simulink library "UXFD_Lib"  (R2016b)
settings: Solver=ode45  StartTime=0.0  StopTime=10.0  RelTol=1e-3  EnableMultiTasking=on
undefined symbols (not defined in the file): BreakpointData, BreakpointData1, BreakpointData2, BreakpointData_One_A, BreakpointData_Two_A, E2E_P01DataIDMode, E2E_P01ReceiverStatusType, EnumClass, iBit, initalValue, No_Runnable_Period, ObB_EidBsgStDerat_C, p_OVERRIDE_MASTER_SWITCH, SlDemoSign, SwitchOff_P, SwitchOn_P, Table, TableData_M, VCCTi33, VSysD_FidVehDerat1_C
libraries: simulink x28, CCMLib x11, UXFD_Lib x8, canmsglib x2, PTCC_Lib x1, hdlsllib x1
(part 4 of 7)

== system UXFD_Lib/Standard/Discrete dynamics ==
  note: Hystresis filter
  note: Bumpless transfer
  note: Unit delay
  note: Discrete
      | derivate
  note: Rate limiter
  note: First order filters (VCC)
  note: Second order filters(VCC)
  BumplessRateTransfer : Subsystem  mask(VCC_BumplessTransferRate_1.0){}
      mask help:
      | Makes a bumpless rate transfer from u2  to u1
      | when s goes from 0 to 1. It is very important that
      |  the Trig signal assumes the values <= 0 and >= 1.
      | The transfer happens during a time controlled by a
      | filter with a time constant that can be calibrated.
      settings: CopyFcn=set_param(gcbh,'ShowName','off');
      mask Display:
      | plot([0.2 1], [0.2 0.2]);
      | plot([0.2 0.3], [0.22 0.22]);
      | plot([0.7 1], [0.78 0.78]);
      | plot([0.2 1], [0.8 0.8]);
      | plot([0.7 1], [0.78 0.78]);
      | plot([0.3 0.7],[0.22, 0.78])
      | plot([0.38, 0.5, 0.52], [0.46, 0.5, 0.37])
  BumplessTransfer : Subsystem  mask(GL_BumplessTransferFilter_1.0){}
      mask help:
      | Makes a bumpless transfer from u2  to u1
      | when s goes from 0 to 1. It is very important that
      |  the Trig signal assumes the values <= 0 and >= 1.
      | The transfer happens during a time controlled by a
      | filter with a time constant that can be calibrated.
      mask init:
      | set_param(gcb,'LinkStatus','none');
      settings: CopyFcn=set_param(gcbh,'ShowName','off');
      mask Display:
      | plot([0.15 1], [0.2 0.2]);
      | plot([0.15 1], [0.8 0.8]);
      | plot([0.00 0.50 1.00 1.50 2.00 2.50 3.00 ]/3*0.7+0.3, ...
      |      [0.20 0.52 0.67 0.74 0.77 0.79 0.79]);
      | 
      | plot([0.28, 0.4, 0.47], [0.48, 0.5, 0.42])
  DLPF1_pole_v2 : Subsystem  mask(GL_DiscreteDerivative_1.0){}
      mask help:
      | Discrete derivative and low-pass filter. Corresponding analogue transfer function:
      |   s / (1 + tc * s)
      mask init:
      | set_param(gcb,'LinkStatus','none');
      settings: CopyFcn=set_param(gcbh,'ShowName','off');
      mask Display:
      | plot([0.35, 0.9], [0, 0], [0.35, 0.35], [0, 1])
      | plot(0.35:0.55/10:0.9,  1- [0 0.39 0.63 0.78 0.86 0.92 0.95 0.97 0.98 0.99 0.99])
  FirstOrderFilter : Subsystem  mask(VCC_FirstOrderFilter_1.0){}
      mask help: Discrete low-pass filter. Corresponding analogue transfer function: 1 / (1 + tc * s)
      settings: CopyFcn=set_param(gcbh,'ShowName','on');
      mask Display:
      | plot([0.35, 0.9], [0, 0], [0.35, 0.35], [0, 1])
      | plot(0.35:0.55/10:0.9,   [0 0.39 0.63 0.78 0.86 0.92 0.95 0.98 0.99 0.99 0.99])
  FirstOrderFilter1 : Subsystem  mask(VCC_FirstOrderFilterExtraFeat_1.0){}
      mask help:
      | Discrete low-pass filter. Corresponding analogue transfer function: 1 / (1 + tc * s)
      |
      | Parameters:
      | Error - An output which shows the difference between the input and output signal values
      | Different increase and decrease tc -
      | Reset - Sets the output value = rv when r = 1
      settings: CopyFcn=set_param(gcbh,'ShowName','on');
      mask Display:
      | plot([0.35, 0.9], [0, 0], [0.35, 0.35], [0, 1])
      | plot(0.35:0.55/10:0.9,   [0 0.39 0.63 0.78 0.86 0.92 0.95 0.98 0.99 0.99 0.99])
  HysteresisFilter : Subsystem  mask(GL_HysteresisFilter_1.0){}
      mask help:
      | Filter to avoid occilation during low slipp
      | when converter character is steep
      mask init:
      | set_param(gcb,'LinkStatus','none');
      settings: CopyFcn=set_param(gcbh,'ShowName','off');
      mask Display:
      | text(0.1, 0.8, 'u');
      | text(0.1, 0.3, 'h');
      | plot([0.3, 0.6, 0.9], [0.1, 0.1, 0.9]);
      | plot([0.3, 0.6, 0.9], [0.1, 0.9, 0.9]);
      | plot([0.4, 0.55], [0.4, 0.4]);
      | plot([0.7, 0.84], [0.7, 0.7]);
  LPF1_discreteReset : Subsystem  Description=|  mask(PAG_FirstOrder_Smoothing_Filter_Reset_LV1.8_BV5){OpenTL=Select block:, OutputLineName=}
      | Purpose Use the block to implement a discrete low pass filter.
      | 
      | When the input signal r is TRUE the output will assume the
      | value of the input signal. This is used to set initial values of
      | the filter.
      | 
      | Difference to Simulink and justification
      | Additional block to perform special feature for ECM implementation
      | in a standard manner. Block name hidden, since icon clearly conveys
      | meaning and name adds unnecessary clutter to the page.
      mask prompts: OpenTL "Open Target Link dialog"; OutputLineName "Output line name"
      mask help:
      | Discrete first order low pass filter. Discrete transfer function:
      | y(k)=a*y(k-1)+(1-a)*u(k)
      | When the input signal r is TRUE the output will assume the
      | value of the input signal. This is used to set initial values of
      | the filter.
      mask init:
      | %% Reset the opendialog popupvalue
      | Values=get_param(gcbh,'maskvalues');
      | Values{1}='Select block:';
      | set_param(gcbh,'maskvalues',Values);
      | 
      | %Set the line name, 
      | CurrentBlock=gcbh;
      | %Find the output variable block
      | while strcmp(get_param(CurrentBlock,'blocktype'),'SubSystem')
      |     Tmp=get_param(find_system(CurrentBlock,'lookundermasks','on','searchdepth',1,'blocktype','Outport','Port','1'),'linehandles');
      |     CurrentBlock=get_param(Tmp.Inport,'srcblockhandle');
      | end
      | set_param(Tmp.Inport,'name',get_param(gcbh,'OutputLineName'));
      | 
      | 
      | %% Adjust the propagated output line name
      | Tmp=get_param(gcbh,'linehandles');
      | OutputLine=Tmp.Outport;
      | if OutputLine~=-1
      |     
      |     if isempty(get_param(gcbh,'OutputLineName'))
      |         set(OutputLine,'signalPropagation','off')
      |         set(OutputLine,'name','')
      |     else
      |         set(OutputLine,'name',['<' get_param(gcbh,'OutputLineName') '>'])
      |     end
      | end
      settings: CopyFcn=set_param(gcbh,'ShowName','on');
      mask TypeOptions OpenTL: Select block: | Output variable
      mask Callback OpenTL:
      | if strcmp(get_param(gcbh,'OpenTL'),'Output variable')
      |     BlockType='SubSystem';
      |     OutputVariableBlock=gcbh;
      |     while strcmp(BlockType,'SubSystem');
      |     Tmp=get_param(find_system(OutputVariableBlock,'lookundermasks','on','searchdepth',1,'blocktype','Outport','Port','1'),'linehandles');
      |     OutputVariableBlock=get_param(Tmp.Inport,'srcblockhandle');
      |     BlockType=get_param(OutputVariableBlock,'blocktype');
      |     end
      | 
      |     MaskType=get_param(OutputVariableBlock,'masktype');
      |     if strmatch('TL',MaskType)
      | 
      |         if ismember(MaskType,{'TL_Sum','TL_Product'})
      |             MaskName='tl_sumprod_dlg';
      |         elseif ismember(MaskType,{'TL_LogicalOperator','TL_RelationalOperator'})
      |             MaskName='tl_rel_dlg';
      |         elseif strcmp(MaskType,'TL_MinMax')
      |             MaskName='tl_minmax_dlg';
      |         elseif strcmp(MaskType,'TL_Gain')
      |             MaskName='tl_gain_dlg';
      |         elseif strcmp(MaskType,'TL_Switch')
      |             MaskName='tl_switch_dlg';
      |         end
      | 
      |         dstabdlg('create',MaskName,OutputVariableBlock);
      |     end
      | end
      mask Display:
      | plot([0.3, 1], [0, 0], [0.3, 0.3], [0, 1])
      | plot([0 0.1 0.1 0.2 0.2 0.3 0.3 0.4 0.4 0.5 0.5 0.6 0.6 0.7 0.7 0.8 0.8 0.9 0.9 1 1]*0.7+0.3, [ 0 0 0.39 0.39 0.63 0.63 0.78 0.78 0.86 0.86 0.92 0.92 0.95 0.95 0.97 0.97 0.98 0.98 0.99 0.99 0.99])
  LPF2_discrete : Subsystem  mask(PAG_SecondOrder_Discrete_Filter_LV1.8_BV3){OpenTL=Select block:, OutputLineName=}
      mask prompts: OpenTL "Open Target Link dialog"; OutputLineName "Output line name"
      mask help:
      | Discrete  filter.
      |
      | y(k) = -a1 y(k-1) - a2 y(k-2) + b0 u(k) + b1 u(k-1) + b2 u(k-2)
      mask init: same as UXFD_Lib/Standard/Discrete dynamics/LPF1_discreteReset
      settings: CopyFcn=set_param(gcbh,'ShowName','off');
      mask TypeOptions OpenTL: Select block: | Output variable
      mask Callback OpenTL:
      | if strcmp(get_param(gcbh,'OpenTL'),'Output variable')
      |     BlockType='SubSystem';
      |     OutputVariableBlock=gcbh;
      |     while strcmp(BlockType,'SubSystem');
      |     Tmp=get_param(find_system(OutputVariableBlock,'lookundermasks','on','searchdepth',1,'blocktype','Outport','Port','1'),'linehandles');
      |     OutputVariableBlock=get_param(Tmp.Inport,'srcblockhandle');
      |     BlockType=get_param(OutputVariableBlock,'blocktype');
      |     end
      | 
      |     MaskType=get_param(OutputVariableBlock,'masktype');
      |     if strmatch('TL',MaskType)
      | 
      |         if ismember(MaskType,{'TL_Sum','TL_Product'})
      |             MaskName='tl_sumprod_dlg';
      |         elseif ismember(MaskType,{'TL_LogicalOperator','TL_RelationalOperator'})
      |             MaskName='tl_rel_dlg';
      |         elseif strcmp(MaskType,'TL_MinMax')
      |             MaskName='tl_minmax_dlg';
      |         elseif strcmp(MaskType,'TL_Gain')
      |             MaskName='tl_gain_dlg';
      |         elseif strcmp(MaskType,'TL_Switch')
      |             MaskName='tl_switch_dlg';
      |         end
      | 
      |         dstabdlg('create',MaskName,OutputVariableBlock);
      |     end
      | end
      mask Display:
      | plot([0.45, 1], [0, 0], [0.45, 0.45], [0, 1])
      | plot([0 0.1 0.1 0.2 0.2 0.3 0.3 0.4 0.4 0.5 0.5 0.6 0.6 0.7 0.7 0.8 0.8 0.9 0.9 1 1]*0.55+0.45, [ 0 0 0.39 0.39 0.63 0.63 0.78 0.78 0.86 0.86 0.92 0.92 0.95 0.95 0.97 0.97 0.98 0.98 0.99 0.99 0.99])
  LPF2_omega : Subsystem  mask(PAG_SecondOrder_Filter_LV1.8_BV4){OpenTL=Select block:, OutputLineName=}
      mask prompts: OpenTL "Open Target Link dialog"; OutputLineName "Output line name"
      mask help:
      | An Euler discretization of a filter with transfer function
      |                          2
      |                       w
      | G(s) = -----------------------------
      |              2                     2
      |            s  + 2 w z s + w
      mask init: same as UXFD_Lib/Standard/Discrete dynamics/LPF1_discreteReset
      settings: CopyFcn=set_param(gcbh,'ShowName','off');
      mask TypeOptions OpenTL: Select block: | Output variable
      mask Callback OpenTL:
      | if strcmp(get_param(gcbh,'OpenTL'),'Output variable')
      |     BlockType='SubSystem';
      |     OutputVariableBlock=gcbh;
      |     while strcmp(BlockType,'SubSystem');
      |     Tmp=get_param(find_system(OutputVariableBlock,'lookundermasks','on','searchdepth',1,'blocktype','Outport','Port','1'),'linehandles');
      |     OutputVariableBlock=get_param(Tmp.Inport,'srcblockhandle');
      |     BlockType=get_param(OutputVariableBlock,'blocktype');
      |     end
      | 
      |     MaskType=get_param(OutputVariableBlock,'masktype');
      |     if strmatch('TL',MaskType)
      | 
      |         if ismember(MaskType,{'TL_Sum','TL_Product'})
      |             MaskName='tl_sumprod_dlg';
      |         elseif ismember(MaskType,{'TL_LogicalOperator','TL_RelationalOperator'})
      |             MaskName='tl_rel_dlg';
      |         elseif strcmp(MaskType,'TL_MinMax')
      |             MaskName='tl_minmax_dlg';
      |         elseif strcmp(MaskType,'TL_Gain')
      |             MaskName='tl_gain_dlg';
      |         elseif strcmp(MaskType,'TL_Switch')
      |             MaskName='tl_switch_dlg';
      |         end
      | 
      |         dstabdlg('create',MaskName,OutputVariableBlock);
      |     end
      | end
      mask Display:
      | plot([0.45, 0.9], [0, 0], [0.45, 0.45], [0, 1])
      | plot(0.45:0.45/10:0.9,   [ 0 0.05 0.1 0.8 1.0 0.95 0.85 0.9 0.95 0.92 0.9 ])
  RateLimit : Subsystem  mask(GL_RateLimiter_1.0){}
      mask help: Rate limiter. Limits the derivative of the input signal to the input value d.
      mask init:
      | set_param(gcb,'LinkStatus','none');
      settings: CopyFcn=set_param(gcbh,'ShowName','off');
      mask Display:
      | plot([0.35, 0.55, 0.55, 1.0], [0, 0, 1, 1])
      | plot([0.35, 0.55, 0.8, 1.0], [0, 0, 1, 1])
  RateLimit1 : Subsystem  mask(GL_RateLimiterExtraFeat_1.0){}
      mask help:
      | Rate limiter. Limits the derivative of the input signal to the input value d.
      |
      | Parameters:
      | Different increase and decrease rate -
      | Reset - Sets the output value = rv when r = 1
      mask init:
      | set_param(gcb,'LinkStatus','none');
      settings: CopyFcn=set_param(gcbh,'ShowName','off');
      mask Display:
      | plot([0.35, 0.55, 0.55, 1.0], [0, 0, 1, 1])
      | plot([0.35, 0.55, 0.8, 1.0], [0, 0, 1, 1])
  Unit Delay : UnitDelay  SampleTime=-1
      settings: CopyFcn=set_param(gcbh,'ShowName','off');
  xbackground1 : Subsystem
      settings: CopyFcn=set_param(gcbh,'ShowName','off');
      mask Display: disp(' ')
  xbackground2 : Subsystem
      settings: CopyFcn=set_param(gcbh,'ShowName','off');
      mask Display: disp(' ')
  xbackground3 : Subsystem
      settings: CopyFcn=set_param(gcbh,'ShowName','off');
      mask Display: disp(' ')
  xbackground4 : Subsystem
      settings: CopyFcn=set_param(gcbh,'ShowName','off');
      mask Display: disp(' ')
  xbackground5 : Subsystem
      settings: CopyFcn=set_param(gcbh,'ShowName','off');
      mask Display: disp(' ')
  xbackground6 : Subsystem
      settings: CopyFcn=set_param(gcbh,'ShowName','off');
      mask Display: disp(' ')
  xbackground7 : Subsystem
      settings: CopyFcn=set_param(gcbh,'ShowName','off');
      mask Display: disp(' ')

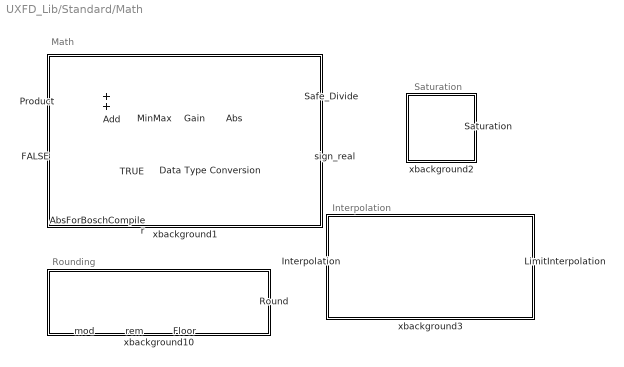
== system UXFD_Lib/Standard/Math ==
  note: Interpolation
  note: Rounding
  note: Math
  note: Saturation
  Abs : Abs
      settings: CopyFcn=set_param(gcbh,'ShowName','off');
  AbsForBoschCompiler : Subsystem  mask(VCC_Abs_1.0){}
      mask help: y=|u|
      mask Display: disp('|u|')
  Add : Sum
      settings: CopyFcn=set_param(gcbh,'ShowName','off');
  Data Type Conversion : DataTypeConversion
      settings: CopyFcn=set_param(gcbh,'ShowName','off');
  FALSE : Constant  ClipboardFcn="href=\"http://183.136.146.131:8080/redmine/my/page\";"  Value=false
      settings: CopyFcn=set_param(gcbh,'ShowName','off');  OpenFcn="href=\"http://183.136.146.131:8080/redmine/my/page\";"
  Floor : Subsystem  mask(GL_Floor){}
      mask help: Floor block rounds the input variable to the nearest integer towards minus infinity.
      settings: CopyFcn=set_param(gcbh,'ShowName','off');
      mask Display: text(0.1,0.5, 'Floor')
  Gain : Gain
      settings: CopyFcn=set_param(gcbh,'ShowName','off');
  Interpolation : Subsystem  mask(GL_Interpolation_1.0){}
      mask help: Linear interpolation. The output is given by y=k(u-x1)+y1, where k=(y2-y1)/(x2-x1)
      settings: CopyFcn=set_param(gcbh,'ShowName','on');
      mask Display:
      | plot([0.2, 0.9], [0.2, 0.2]);
      | plot([0.2, 0.2], [0.2, 0.9]);
      | plot([0.4,  0.6], [0.25, 0.85]);
      | text(0.40, 0.27, '(x1, y1)');
      | text(0.50, 0.88, '(x2, y2)');
  LimitInterpolation : Subsystem  mask(GL_LimitInterpolation_1.0){}
      mask help:
      | Interpolation with limitations.  The output is given by  y=k(u-x1)+y1, where k=(y2-y1)/(x2-x1)
      | The output value is also limited to the interval  y1 < y < y2.
      settings: CopyFcn=set_param(gcbh,'ShowName','on');
      mask Display:
      | plot([0.2, 0.9], [0.2, 0.2]);
      | plot([0.2, 0.2], [0.2, 0.9]);
      | plot([0.25, 0.4,  0.6, 0.85], [0.25, 0.25, 0.85, 0.85]);
      | text(0.40, 0.27, '(x1,  y1)');
      | text(0.50, 0.88, '(x2,  y2)');
  MinMax : MinMax
      settings: CopyFcn=set_param(gcbh,'ShowName','off');
  Product : Product
      settings: CopyFcn=set_param(gcbh,'ShowName','off');
  Round : Subsystem  mask(GL_Round){}
      mask help: Rounds to nearest integer
      settings: CopyFcn=set_param(gcbh,'ShowName','off');
      mask Display: text(0.1,0.5, 'Round')
  Safe_Divide : Subsystem  mask(GL_SafeDivide_1.0){}
      mask help:
      | Safe Divide, prevents division by zero.
      |
      | if abs(denominator) > eps then
      |     output = numerator / denominator
      | else
      |     output = numerator / eps
      |
      | Attention!
      | Use this block only when there is a risk for division by zero.
      mask Display:
      | port_label('input', 1, 'x')
      | port_label('input', 2, '÷')
      | port_label('input', 3, 'eps')
  Saturation : Subsystem  mask(GL_Saturation_1.0){}
      mask help:
      | If input_1 > input_2
      |   output = input_2
      | elseif input_1 < input_3
      |   output = input_3
      | else
      |   output = input_1
      |
      | Note that if the lower limit is set above the upper limit, the output will take the value of the input to the lower limit port.
      settings: CopyFcn=set_param(gcbh,'ShowName','off');
      mask Display: plot([0.3, 0.5, 0.7, 0.9], [0, 0, 1, 1])
  TRUE : Constant  Value=true
      settings: CopyFcn=set_param(gcbh,'ShowName','off');
  mod : Subsystem  mask(GL_Mod_1.0){}
      mask help: Signed remainder after division.
      settings: CopyFcn=set_param(gcbh,'ShowName','off');
      mask Display: disp('mod')
  rem : Subsystem  mask(GL_Rem_1.0){}
      mask help: Remainder after division.
      settings: CopyFcn=set_param(gcbh,'ShowName','off');
      mask Display: disp('rem')
  sign_real : Subsystem
      mask Display:
      | text(0.18, 0.275, '-1');
      | text(0.75, 0.75, '1');
      | text(0.55, 0.42, '0');
      | plot([0.25, 0.5, 0.5, 0.75],[0.25, 0.25, 0.75, 0.75])
      | plot([0,1],[0.5, 0.5])
      | plot([0.5,0.5],[0,1])
  xbackground1 : Subsystem
      mask Display: disp(' ')
  xbackground10 : Subsystem
      mask Display: disp(' ')
  xbackground2 : Subsystem
      mask Display: disp(' ')
  xbackground3 : Subsystem
      mask Display: disp(' ')

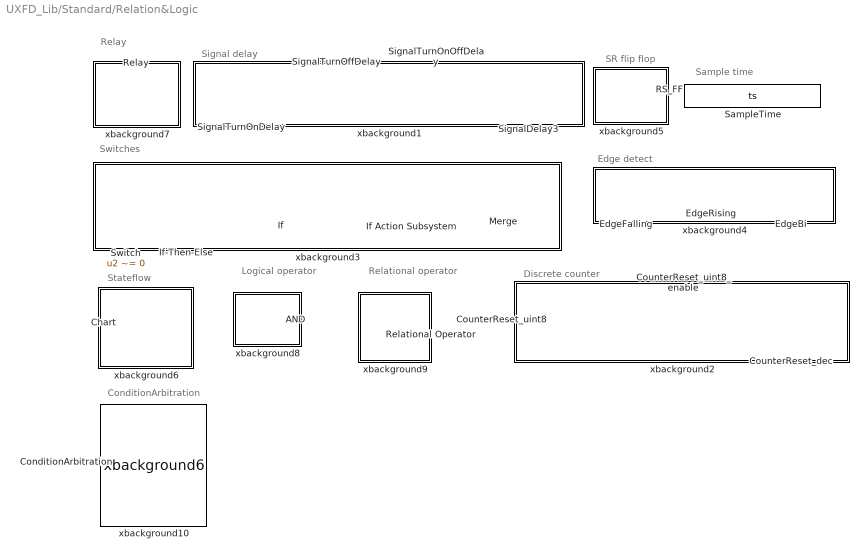
== system UXFD_Lib/Standard/Relation&Logic ==
  note: Relay
  note: Signal delay
  note: Edge detect
  note: Switches
  note: SR flip flop
  note: Stateflow
  note: Logical
      | operator
  note: Relational
      |  operator
  note: Discrete counter
  note: Sample time
  note: ConditionArbitration
  AND : Logic  AllPortsSameDT=off  OutDataTypeStr=boolean
      settings: CopyFcn=set_param(gcbh,'ShowName','off');
  Chart : Stateflow chart  TreatAsAtomicUnit=on
      settings: CopyFcn=set_param(gcbh,'ShowName','off');
  ConditionArbitration : Subsystem  mask(ConditionArbitration){}
      mask help:
      | If Condition1 == Condition2 == 0
      |   Val_0_0 send out
      | elseif Condition1== 0 && Condition2 == 1
      |   Val_0_1 send out
      | elseif Condition1== 1 && Condition2 == 0
      |   Val_1_0 send out
      | else
      |   Val_1_1 send out
      mask Display:
      | port_label('input', 1, 'Condition1');
      | port_label('input', 2, 'Condition2');
      | port_label('input', 3, '0 0');
      | port_label('input', 4, '0 1');
      | port_label('input', 5, '1 0');
      | port_label('input', 6, '1 1');
      | port_label('output', 1, 'out');
  CounterReset_dec : Subsystem  mask(GL_DecreseCounterEnableReset_1.0){}
      mask help:
      | Resetable counter.
      |
      | If r = 1 the counter resets to rv.
      | If r = 0 the block adds/subtracts inc/dec to the output each sample.
      |
      | To count time let inc/dec = sample_time
      | To count samples let inc/dec = 1
      |
      | Enable: Enables the counter if e = 1
      | Dec: Counts down instead of up. Stops counting when output = 0
      settings: CopyFcn=set_param(gcbh,'ShowName','off');
      mask Display:
      | plot([ 0.5 1 1 2 2 3 3 4 4 5 5 6 6 7 7]/14+0.4, ...
      |        [ 0 0 4 4 3 3 2 2 1 1 0 0 0 0 0]/5+0.1)
  CounterReset_uint8 : Subsystem  mask(GL_CounterReset_1.0){}
      mask help:
      | Resetable counter.
      |
      | If r = 1 the counter resets to rv.
      | If r = 0 the block adds/subtracts inc/dec to the output each sample.
      |
      | To count time let inc/dec = sample_time
      | To count samples let inc/dec = 1
      |
      | Enable: Enables the counter if e = 1
      | Dec: Counts down instead of up. Stops counting when output = 0
      settings: CopyFcn=set_param(gcbh,'ShowName','off');
      mask Display: plot([0 1 1 2 2 3 3 4 4 5]/14+0.4, [0 0 1 1 2 2 3 3 4 4]/5+0.1)
  CounterReset_uint8_enable : Subsystem  mask(VCC_CounterEnableReset_1.0){}
      mask help:
      | Resetable counter.
      |
      | If r = 1 the counter resets to rv.
      | If r = 0 the block adds/subtracts inc/dec to the output each sample.
      |
      | To count time let inc/dec = sample_time
      | To count samples let inc/dec = 1
      |
      | Enable: Enables the counter if e = 1
      | Dec: Counts down instead of up. Stops counting when output = 0
      settings: CopyFcn=set_param(gcbh,'ShowName','off');
      mask Display: plot([0 1 1 2 2 3 3 4 4 5]/14+0.4, [0 0 1 1 2 2 3 3 4 4]/5+0.1)
  EdgeBi : Subsystem  mask(GL_EdgeDetectEither_1.0){}
      mask help: Output is 1 of negative or positive edge is detected, otherwise its 0.
      settings: CopyFcn=set_param(gcbh,'ShowName','off');
      mask Display:
      | plot([0 0.5 0.5 1.5 1.5 2], [0 0 1 1 0 0])
      | 
      | patch([0 1 0.5 0], [0.25 0.25 0.85 0.25])
      | patch([1 2 1.5 1], [0.75 0.75 0.15 0.75])
  EdgeFalling : Subsystem  mask(GL_EdgeDetectNegative_1.0){}
      mask help: Output is 1 of negative edge is detected, otherwise its 0.
      settings: CopyFcn=set_param(gcbh,'ShowName','off');
      mask Display:
      | plot([0 0.5 0.5 1.5 1.5 2], [0 0 1 1 0 0])
      | patch([1 2 1.5 1], [0.75 0.75 0.15 0.75])
  EdgeRising : Subsystem  mask(GL_EdgeDetectPositive_1.0){}
      mask help: Output is 1 of positive edge is detected, otherwise its 0.
      settings: CopyFcn=set_param(gcbh,'ShowName','off');
      mask Display:
      | plot([0 0.5 0.5 1.5 1.5 2], [0 0 1 1 0 0])
      | 
      | patch([0 1 0.5 0], [0.25 0.25 0.85 0.25])
  If : If
      settings: CopyFcn=set_param(gcbh,'ShowName','off');
  If Action Subsystem : Subsystem  TreatAsAtomicUnit=on
      settings: CopyFcn=|
      | set_param(gcbh,'ShowName','off');
      | set_param(gcbh,'LinkStatus','none');
  If-Then-Else : Subsystem
      mask Display:
      | port_label('input',1,'If')
      | port_label('input',2,'Then')
      | port_label('input',3,'Else')
  Merge : Merge
      settings: CopyFcn=set_param(gcbh,'ShowName','off');
  RS_FF : Subsystem  mask(GL_SRFlipFlop_1.0){}
      mask help:
      | Set/Reset flip flop.
      |
      |   R   S   Q
      |   1   X   0            (X :  0 or 1)
      |   0   1   1            (P:   keeps previous value)
      |   0   0   P
      settings: CopyFcn=set_param(gcbh,'ShowName','off');
  Relational Operator : RelationalOperator  Operator=<=  OutDataTypeStr=boolean  RndMeth=Nearest
      settings: CopyFcn=set_param(gcbh,'ShowName','off');
  Relay : Subsystem  mask(GL_Relay_1.0){}
      mask help: Output 1 or 0 ('on' or 'off') by comparing the first input to the thresholds specified by thesecond and third input. The switch on point is specified by the second input and the switch off point is specified by the third input. If the second input becomes less then the third input the relay switch off. The on/off state of the relay is not affected by input between the upper and lower limits.
      settings: CopyFcn=set_param(gcbh,'ShowName','off');
      mask Display: plot( [0.4 0.8 0.8], [0.05  0.05 0.8], [0.6 0.6 0.9], [0.05 0.8 0.8])
  SampleTime : DataStoreMemory  DataStoreName=ts  InitialValue=0.01  ShowAdditionalParam=off  OutDataTypeStr=single  mask(DataStoreMemory){data={'output',{'description',['Sample time'],'name','ts','class','STATIC_MACRO','type','Float32','unit','s'},'date',735300.29223179398}}
      settings: CopyFcn=set_param(gcbh,'ShowName','off');
      mask Display: plot([-0.05, 1.05, NaN, -0.05, 1.05],[.01, .01, NaN, .99, .99])
  SignalDelay3 : Subsystem  mask(GL_SignalDelayEither_1.0){}
      mask help: Signal delay. Delays a logical change the time td. The output signal will not change unless the input signal keeps its value during the time td.
      settings: CopyFcn=set_param(gcbh,'ShowName','off');
      mask Display:
      | plot([0.4 0.7 0.7 0.8], [0.3 0.3 0.7 0.7]+0.3)
      | plot([0.4 0.7 0.7 0.8], [0.7 0.7 0.3 0.3]-0.3)
  SignalTurnOffDelay : Subsystem  mask(VCC_SignalDelayNegative_1.0){}
      mask help: Signal delay. Delays a negative logical change the time td. The output signal will not change unless the input signal keeps its value during the time td.
      mask init:
      | set_param(gcb,'LinkStatus','none');
      settings: CopyFcn=set_param(gcbh,'ShowName','off');
      mask Display: plot([0.4 0.7 0.7 0.8], [0.7 0.7 0.3 0.3])
  SignalTurnOnDelay : Subsystem  mask(GL_SignalDelayPositive_1.0){}
      mask help: Signal delay. Delays a positive logical change the time td. The output signal will not change unless the input signal keeps its value during the time td.
      settings: CopyFcn=set_param(gcbh,'ShowName','off');
      mask Display: plot([0.4 0.7 0.7 0.8], [0.3 0.3 0.7 0.7])
  SignalTurnOnOffDelay : Subsystem  mask(GL_SignalDelayEither_1.0){}
      mask help: Signal delay. Delays a logical change the time td. The output signal will not change unless the input signal keeps its value during the time td.
      settings: CopyFcn=set_param(gcbh,'ShowName','off');
      mask Display:
      | plot([0.4 0.7 0.7 0.8], [0.3 0.3 0.7 0.7]+0.3)
      | plot([0.4 0.7 0.7 0.8], [0.7 0.7 0.3 0.3]-0.3)
  Switch : Switch  Criteria=u2 ~= 0  OutDataTypeStr=Inherit: Inherit via back propagation  RndMeth=Round  SaturateOnIntegerOverflow=on  InputSameDT=on
      mask init:
      | set_param(gcb, 'LinkStatus', 'none');
      | % 这句的使用场景：
      | % 当模型没有这句时，模型传递给没有模型库的人员会出现红色的错误框
      | % 没有模型库的使用者不能查看此模块
      settings: CopyFcn=set_param(gcb,'showname','off');
      mask Display:
      | plot([0.54 0.65],[0.92 0.92])
      | plot([0.6 0.6],[0.84 0.92])
      | 
      | plot([0.54 0.54],[0.05 0.14])
      | plot([0.54 0.65],[0.14 0.14])
      | plot([0.54 0.625],[0.08 0.08])
  xbackground1 : Subsystem
      mask Display: disp(' ')
  xbackground10 : UXFD_Lib/Standard/Relation&Logic/xbackground6  SystemSampleTime=-1
  xbackground2 : Subsystem
      mask Display: disp(' ')
  xbackground3 : Subsystem
      mask Display: disp(' ')
  xbackground4 : Subsystem
      mask Display: disp(' ')
  xbackground5 : Subsystem
      mask Display: disp(' ')
  xbackground6 : Subsystem
      mask Display: disp(' ')
  xbackground7 : Subsystem
      mask Display: disp(' ')
  xbackground8 : Subsystem
      mask Display: disp(' ')
  xbackground9 : Subsystem
      mask Display: disp(' ')

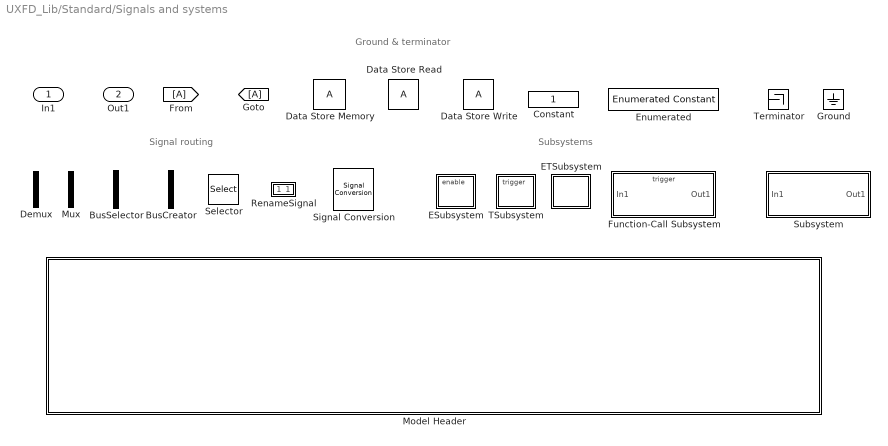
== system UXFD_Lib/Standard/Signals and systems ==
  note: Subsystems
  note: Ground & terminator
  note: Signal routing
  In1 : Inport
  BusCreator : BusCreator  Inputs=2
      settings: CopyFcn=set_param(gcbh,'ShowName','off');
  BusSelector : BusSelector  OutputSignals=signal1,signal2
      settings: CopyFcn=set_param(gcbh,'ShowName','off');
  Constant : Constant  OutDataTypeStr=Inherit: Inherit via back propagation
      settings: CopyFcn=set_param(gcbh,'ShowName','off');
  Data Store Memory : DataStoreMemory  ReadBeforeWriteMsg=warning  WriteAfterWriteMsg=warning  WriteAfterReadMsg=warning  ShowAdditionalParam=off
      settings: CopyFcn=set_param(gcbh,'ShowName','off');
  Data Store Read : DataStoreRead
      settings: CopyFcn=set_param(gcbh,'ShowName','off');
  Data Store Write : DataStoreWrite
      settings: CopyFcn=set_param(gcbh,'ShowName','off');
  Demux : Demux  Outputs=3
      settings: CopyFcn=set_param(gcbh,'ShowName','off');
  ESubsystem : Subsystem  TreatAsAtomicUnit=on
      mask init:
      | set_param(gcb, 'LinkStatus', 'none');
      mask Display: disp(' ');
  ETSubsystem : Subsystem  TreatAsAtomicUnit=on
      mask init:
      | set_param(gcb, 'LinkStatus', 'none');
      mask Display: disp(' ');
  Enumerated : simulink/Sources/Enumerated Constant  OutDataTypeStr=Enum: SlDemoSign  Value=SlDemoSign.Positive  SampleTime=inf
  Function-Call Subsystem : Subsystem  TreatAsAtomicUnit=on
      mask init:
      | set_param(gcb, 'LinkStatus', 'none');
  Ground : Ground
      settings: CopyFcn=set_param(gcbh,'ShowName','off');
  Model Header : Subsystem  mask(ModelHeader){prj='48V XXXXX', desc='Model Description', ver='V1.0.1', date='2017. 10. 12', rev='0', author=' '}
      mask prompts: prj "Project"; desc "Description"; ver "Version"
      mask init:
      | set_param(gcb, 'LinkStatus', 'none');
      settings: CopyFcn=set_param(gcbh,'ShowName','off');
      mask Display:
      | plot([0 0 1 1 0],[0.03 1 1 0.03 0.03])
      | plot([0 1],[0.4 0.4])
      | plot([0.5 0.5],[0.4 1])
      | plot([0.59 0.59],[0.4 1])
      | plot([0.5 1],[0.8 0.8])
      | plot([0.5 1],[0.6 0.6])
      | plot([0.75 0.75],[0.4 1])
      | plot([0.82 0.82],[0.6 1])
      | plot([0.75 0.75],[0.6 0.8])
      | plot([0.82 0.82],[0.4 0.8])
      | image(imread('geely.png','png'),[0.16 0.43 0.15 0.53])
      | text(0.01,0.34,['\fontsize{14}\fontname{Times}\bfPROPRIETARY AND CONFIDENTIAL:\rm\fontsize{11}\newline\it\fontsize{13}\fontname{Arial}'                 '    The Information Contained In This Model Is The Property Of Geely Automobile Research Institute. All Right Reserved.'                 ],'verticalAlignment','Top','horizontalAlignment','Left','texmode','on');
      | text(0.51,0.96,['\fontsize{14}\fontname{Times}\bfProject:       \rm\fontsize{11}\fontsize{12}' prj],'verticalAlignment','Top','horizontalAlignment','Left','texmode','on');
      | text(0.51,0.77,['\fontsize{14}\fontname{Times}\bfVersion:       \rm\fontsize{11}\fontsize{12}' ver],'verticalAlignment','Top','horizontalAlignment','Left','texmode','on');
      | text(0.51,0.56,['\fontsize{14}\fontname{Times}\bfDate:           \rm\fontsize{11}\fontsize{12}' date],'verticalAlignment','Top','horizontalAlignment','Left','texmode','on');
      | text(0.76,0.56,['\fontsize{14}\fontname{Times}\bfModel:    \rm\fontsize{11}\fontsize{12}' desc],'verticalAlignment','Top','horizontalAlignment','Left','texmode','on');
      | text(0.76,0.77,['\fontsize{14}\fontname{Times}\bfRev:        \rm\fontsize{11}\fontsize{12}' rev],'verticalAlignment','Top','horizontalAlignment','Left','texmode','on');
      | text(0.76,0.96,['\fontsize{14}\fontname{Times}\bfAuthor:    \rm\fontsize{11}\fontsize{12}' author],'verticalAlignment','Top','horizontalAlignment','Left','texmode','on');
  Mux : Mux  Inputs=3
      settings: CopyFcn=set_param(gcbh,'ShowName','off');
  RenameSignal : Subsystem  mask(GL_RenameSignal_1.0){}
      mask help: This block should be used to rename signals.
      mask init:
      | set_param(gcb, 'LinkStatus','none');
      settings: CopyFcn=set_param(gcbh,'ShowName','off');
      mask Display:
      | plot([0,1],[0.5,0.5]);
      | patch([0.2, 0.5, 0.2], [0.0,0.5, 1]);
      | patch([0.6, 0.9, 0.6], [0.0,0.5, 1]);
      | plot([0, 1, 1, 0, 0], [0, 0, 1, 1, 0])
  Selector : Selector  InputPortWidth=3  IndexOptions=Index vector (dialog)  Indices=[1 3]  OutputSizes=1
      settings: CopyFcn=set_param(gcbh,'ShowName','off');
  Signal Conversion : SignalConversion  ConversionOutput=Contiguous copy  OverrideOpt=off
      settings: CopyFcn=set_param(gcbh,'ShowName','off');
  Subsystem : Subsystem
  TSubsystem : Subsystem  TreatAsAtomicUnit=on
      mask init:
      | set_param(gcb, 'LinkStatus', 'none');
      mask Display: disp(' ');
  Terminator : Terminator
      settings: CopyFcn=set_param(gcbh,'ShowName','off');
  Out1 : Outport  Port=2

== system UXFD_Lib/Autosar/E2E_P01Protect/E2E_P01Protect ==
  DataLength : Inport
  DataID : Inport  Port=2
  Vmc_Out_BrkActrCtrlModForMinTqReq : Inport  Port=3
  Vmc_Out_BrkTqGrdtNegMinReq : Inport  Port=4
  Vmc_Out_BrkTqGrdtPosMinReq : Inport  Port=5
  Vmc_Out_BrkTqMinReq : Inport  Port=6
  RollingCounter_In : Inport  Port=7
  CheckSum_In : Inport  Port=8
  BusCreator1 : BusCreator  Inputs=1  OutDataTypeStr=Bus: E2E_P01SenderStateType  NonVirtualBus=on
      settings: CopyFcn=set_param(gcbh,'ShowName','off');  InheritFromInputs=off
  BusSelector : BusSelector  OutputSignals=Counter
      settings: CopyFcn=set_param(gcbh,'ShowName','off');
  Data Type Conversion : DataTypeConversion
  Data_Pack : Subsystem
  E2E_Config : Subsystem
  E2E_P01Protect_S : Subsystem
      mask Display:
      | disp('E2E_P01Protect');
      | port_label('input',1,'ConfigType');
      | port_label('input',2,'SenderStateType');
      | port_label('input',3,'Data_pu8');
      | port_label('output',1,'Std_ReturnType');
  Unit Delay : UnitDelay  SampleTime=-1
  E2E_P01Protect_ReturnType : Outport
  Data_pu8 : Outport  Port=2
  wires:
  BusSelector/1 -> Unit Delay/1  "<Counter>"
  BusCreator1/1 -> E2E_P01Protect_S/2(SenderStateType), BusSelector/1
  Unit Delay/1 -> BusCreator1/1
  E2E_P01Protect_S/1(Std_ReturnType) -> E2E_P01Protect_ReturnType/1
  E2E_Config/1(E2E_P01_Config) -> E2E_P01Protect_S/1(ConfigType)
  DataLength/1 -> E2E_Config/1(DataLength)
  DataID/1 -> E2E_Config/2(DataID)
  Data Type Conversion/1 -> Data_pu8/1, E2E_P01Protect_S/3(Data_pu8)
  Data_Pack/1(Data_pu8) -> Data Type Conversion/1
  Vmc_Out_BrkTqGrdtPosMinReq/1 -> Data_Pack/3(Vmc_Out_BrkTqGrdtPosMinReq)
  Vmc_Out_BrkTqGrdtNegMinReq/1 -> Data_Pack/2(Vmc_Out_BrkTqGrdtNegMinReq)
  Vmc_Out_BrkTqMinReq/1 -> Data_Pack/4(Vmc_Out_BrkTqMinReq)
  Vmc_Out_BrkActrCtrlModForMinTqReq/1 -> Data_Pack/1(Vmc_Out_BrkActrCtrlModForMinTqReq)
  RollingCounter_In/1 -> Data_Pack/5(RollingCounter_In)
  CheckSum_In/1 -> Data_Pack/6(CheckSum_In)

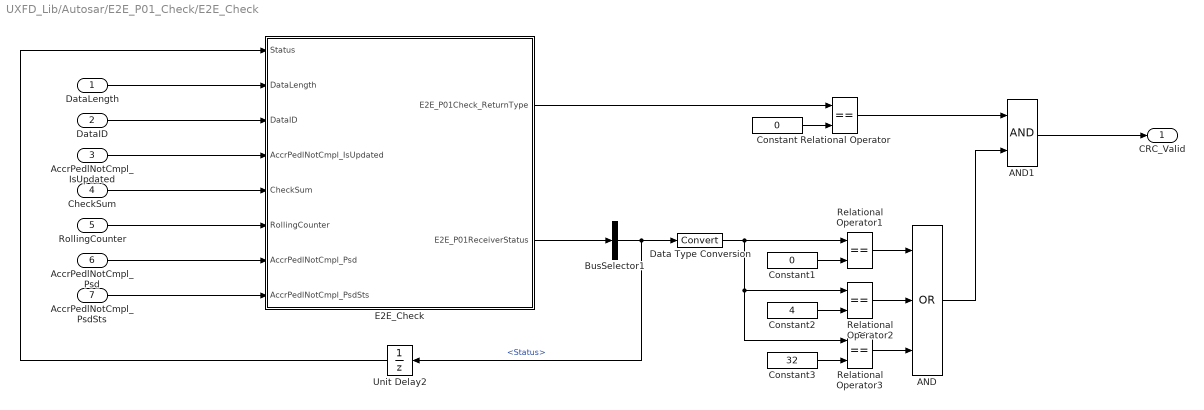
== system UXFD_Lib/Autosar/E2E_P01_Check/E2E_Check ==
  DataLength : Inport
  DataID : Inport  Port=2
  AccrPedlNotCmpl_IsUpdated : Inport  Port=3
  CheckSum : Inport  Port=4
  RollingCounter : Inport  Port=5
  AccrPedlNotCmpl_Psd : Inport  Port=6
  AccrPedlNotCmpl_PsdSts : Inport  Port=7
  AND : Logic  Operator=OR  Inputs=3  AllPortsSameDT=off  OutDataTypeStr=boolean
      settings: CopyFcn=set_param(gcbh,'ShowName','off');
  AND1 : Logic  AllPortsSameDT=off  OutDataTypeStr=boolean
      settings: CopyFcn=set_param(gcbh,'ShowName','off');
  BusSelector1 : BusSelector  OutputSignals=Status
      settings: CopyFcn=set_param(gcbh,'ShowName','off');
  Constant : Constant  Value=0  OutDataTypeStr=Inherit: Inherit via back propagation
      settings: CopyFcn=set_param(gcbh,'ShowName','off');
  Constant1 : Constant  Value=0  OutDataTypeStr=Inherit: Inherit via back propagation
      settings: CopyFcn=set_param(gcbh,'ShowName','off');
  Constant2 : Constant  Value=4  OutDataTypeStr=Inherit: Inherit via back propagation
      settings: CopyFcn=set_param(gcbh,'ShowName','off');
  Constant3 : Constant  Value=32  OutDataTypeStr=Inherit: Inherit via back propagation
      settings: CopyFcn=set_param(gcbh,'ShowName','off');
  Data Type Conversion : DataTypeConversion
  E2E_Check : Subsystem  TreatAsAtomicUnit=on
  Relational Operator{,1..3} (4 alike) : RelationalOperator  Operator===  OutDataTypeStr=boolean  RndMeth=Nearest
      settings: CopyFcn=set_param(gcbh,'ShowName','off');
  Unit Delay2 : UnitDelay  InitialCondition=E2E_P01ReceiverStatusType.E2E_P01STATUS_OK  SampleTime=-1
  CRC_Valid : Outport
  wires:
  BusSelector1/1 -> Data Type Conversion/1, Unit Delay2/1  "<Status>"
  DataLength/1 -> E2E_Check/2(DataLength)
  DataID/1 -> E2E_Check/3(DataID)
  AccrPedlNotCmpl_IsUpdated/1 -> E2E_Check/4(AccrPedlNotCmpl_IsUpdated)
  CheckSum/1 -> E2E_Check/5(CheckSum)
  RollingCounter/1 -> E2E_Check/6(RollingCounter)
  Unit Delay2/1 -> E2E_Check/1(Status)
  E2E_Check/1(E2E_P01Check_ReturnType) -> Relational Operator/1
  E2E_Check/2(E2E_P01ReceiverStatus) -> BusSelector1/1
  Constant/1 -> Relational Operator/2
  Constant1/1 -> Relational Operator1/2
  Constant2/1 -> Relational Operator2/2
  Constant3/1 -> Relational Operator3/2
  Relational Operator1/1 -> AND/1
  Relational Operator3/1 -> AND/3
  Relational Operator2/1 -> AND/2
  AND1/1 -> CRC_Valid/1
  Data Type Conversion/1 -> Relational Operator3/1, Relational Operator2/1, Relational Operator1/1
  AccrPedlNotCmpl_Psd/1 -> E2E_Check/7(AccrPedlNotCmpl_Psd)
  AccrPedlNotCmpl_PsdSts/1 -> E2E_Check/8(AccrPedlNotCmpl_PsdSts)
  Relational Operator/1 -> AND1/1
  AND/1 -> AND1/2

== system UXFD_Lib/CCM/LowPass filter Resettable/Unit Delay Resettable External IC boolean controlled ==
  u : Inport  OutDataTypeStr=dt
  R : Inport  Port=2  OutDataTypeStr=boolean
  IC : Inport  Port=3  OutDataTypeStr=dt
  FixPt Constant : Constant  DisableCoverage=on  Value=false  OutDataTypeStr=boolean  SampleTime=-1
  FixPt Data Type Duplicate1 : DataTypeDuplicate  DisableCoverage=on  NumInputPorts=4
  FixPt Logical Operator : Logic  DisableCoverage=on  Operator=OR  AllPortsSameDT=off  OutDataTypeStr=boolean
  FixPt Unit Delay1 : UnitDelay  DisableCoverage=on  InitialCondition=UnitDelayInitCondition  SampleTime=-1  HasFrameUpgradeWarning=off
  FixPt Unit Delay2 : UnitDelay  DisableCoverage=on  InitialCondition=true  SampleTime=-1
  Init : Switch  Criteria=u2 ~= 0  OutDataTypeStr=Inherit: Inherit via back propagation  ZeroCross=off  SaturateOnIntegerOverflow=on
  Reset : Switch  Criteria=u2 ~= 0  OutDataTypeStr=Inherit: Inherit via back propagation  ZeroCross=off  SaturateOnIntegerOverflow=on
  y : Outport  OutDataTypeStr=dt
  wires:
  FixPt Logical Operator/1 -> Init/2
  FixPt Unit Delay1/1 -> Init/3
  Init/1 -> y/1, FixPt Data Type Duplicate1/1
  FixPt Unit Delay2/1 -> FixPt Logical Operator/2
  FixPt Constant/1 -> FixPt Unit Delay2/1
  R/1 -> FixPt Logical Operator/1, Reset/2
  Reset/1 -> FixPt Unit Delay1/1, FixPt Data Type Duplicate1/2
  u/1 -> Reset/3, FixPt Data Type Duplicate1/4
  IC/1 -> FixPt Data Type Duplicate1/3, Init/1, Reset/1

== system UXFD_Lib/CCM/LowPass filter IC Resettable/Unit Delay Resettable External IC boolean controlled ==
  u : Inport  OutDataTypeStr=dt
  R : Inport  Port=2  OutDataTypeStr=boolean
  IC : Inport  Port=3  OutDataTypeStr=dt
  FixPt Constant : Constant  DisableCoverage=on  Value=false  OutDataTypeStr=boolean  SampleTime=-1
  FixPt Data Type Duplicate1 : DataTypeDuplicate  DisableCoverage=on  NumInputPorts=4
  FixPt Logical Operator : Logic  DisableCoverage=on  Operator=OR  AllPortsSameDT=off  OutDataTypeStr=boolean
  FixPt Unit Delay1 : UnitDelay  DisableCoverage=on  InitialCondition=UnitDelayInitCondition  SampleTime=-1  HasFrameUpgradeWarning=off
  FixPt Unit Delay2 : UnitDelay  DisableCoverage=on  InitialCondition=true  SampleTime=-1
  Init : Switch  Criteria=u2 ~= 0  OutDataTypeStr=Inherit: Inherit via back propagation  ZeroCross=off  SaturateOnIntegerOverflow=on
  Reset : Switch  Criteria=u2 ~= 0  OutDataTypeStr=Inherit: Inherit via back propagation  ZeroCross=off  SaturateOnIntegerOverflow=on
  y : Outport  OutDataTypeStr=dt
  wires:
  IC/1 -> Reset/1, Init/1, FixPt Data Type Duplicate1/3
  u/1 -> FixPt Data Type Duplicate1/4, Reset/3
  Reset/1 -> FixPt Data Type Duplicate1/2, FixPt Unit Delay1/1
  R/1 -> Reset/2, FixPt Logical Operator/1
  FixPt Constant/1 -> FixPt Unit Delay2/1
  FixPt Unit Delay2/1 -> FixPt Logical Operator/2
  Init/1 -> FixPt Data Type Duplicate1/1, y/1
  FixPt Unit Delay1/1 -> Init/3
  FixPt Logical Operator/1 -> Init/2

== system UXFD_Lib/CCM/Rate Limiter Resettable IC/Unit Delay Resettable External IC boolean controlled ==
  u : Inport  OutDataTypeStr=dt
  R : Inport  Port=2  OutDataTypeStr=boolean
  IC : Inport  Port=3  OutDataTypeStr=dt
  FixPt Constant : Constant  DisableCoverage=on  Value=false  OutDataTypeStr=boolean  SampleTime=-1
  FixPt Data Type Duplicate1 : DataTypeDuplicate  DisableCoverage=on  NumInputPorts=4
  FixPt Logical Operator : Logic  DisableCoverage=on  Operator=OR  AllPortsSameDT=off  OutDataTypeStr=boolean
  FixPt Unit Delay1 : UnitDelay  DisableCoverage=on  InitialCondition=UnitDelayInitCondition  SampleTime=-1  HasFrameUpgradeWarning=off
  FixPt Unit Delay2 : UnitDelay  DisableCoverage=on  InitialCondition=true  SampleTime=-1
  Init : Switch  Criteria=u2 ~= 0  OutDataTypeStr=Inherit: Inherit via back propagation  ZeroCross=off  SaturateOnIntegerOverflow=on
  Reset : Switch  Criteria=u2 ~= 0  OutDataTypeStr=Inherit: Inherit via back propagation  ZeroCross=off  SaturateOnIntegerOverflow=on
  y : Outport  OutDataTypeStr=dt
  wires:
  FixPt Logical Operator/1 -> Init/2
  FixPt Unit Delay1/1 -> Init/3
  Init/1 -> y/1, FixPt Data Type Duplicate1/1
  FixPt Unit Delay2/1 -> FixPt Logical Operator/2
  FixPt Constant/1 -> FixPt Unit Delay2/1
  R/1 -> FixPt Logical Operator/1, Reset/2
  Reset/1 -> FixPt Unit Delay1/1, FixPt Data Type Duplicate1/2
  u/1 -> Reset/3, FixPt Data Type Duplicate1/4
  IC/1 -> FixPt Data Type Duplicate1/3, Init/1, Reset/1

== system UXFD_Lib/Custom/CAN/CAN_Receive ==
  In1 : Inport
  In2 : Inport  Port=2
  Return_Value : S-Function  FunctionName=ACTION_CANBSW_RecMsg_S  SFunctionDeploymentMode=off  EnableBusSupport=off
  Out1 : Outport
  wires:
  Return_Value/1 -> Out1/1
  In2/1 -> Return_Value/2
  In1/1 -> Return_Value/1

== system UXFD_Lib/Custom/CAN/CAN_Transmit ==
  In1 : Inport
  In2 : Inport  Port=2
  S-Function : S-Function  FunctionName=ACTION_CANBSW_SndMsg_S  SFunctionDeploymentMode=off  EnableBusSupport=off
  Out1 : Outport
  wires:
  In1/1 -> S-Function/1
  In2/1 -> S-Function/2
  S-Function/1 -> Out1/1

== system UXFD_Lib/Custom/CAN/CanHex2Signed ==
  note: 计算判断条件： 2 n-1 -1
      | 和2^n
  note: 判断输入的BitLength是否（0<u1<=32bit）;
      | 并向下取整。
  hex : Inport
  Add4 : Sum
      settings: CopyFcn=set_param(gcbh,'ShowName','off');
  Constant1 : Constant  Value=BitLength
  Constant5 : Constant  Value=Factor
  Constant6 : Constant  Value=Offset
  If : If  IfExpression=u1 == 1
      settings: CopyFcn=set_param(gcbh,'ShowName','off');
  Merge : Merge
      settings: CopyFcn=set_param(gcbh,'ShowName','off');
  Product : Product  OutDataTypeStr=single
      settings: CopyFcn=set_param(gcbh,'ShowName','off');
  Relational Operator : RelationalOperator  Operator=<  OutDataTypeStr=boolean  RndMeth=Nearest
  condtion : Subsystem
  signal_conditioning : Subsystem
  value<0 : Subsystem  TreatAsAtomicUnit=on
  value>0 : Subsystem  TreatAsAtomicUnit=on
  Out1 : Outport
  wires:
  value>0/1(Out1) -> Merge/2
  [index] -> value<0/2(2^n)
  condtion/2(2^n) -> [index]
  Relational Operator/1 -> If/1
  If/1 -> value<0/Action
  If/2 -> value>0/Action
  hex/1 -> Relational Operator/2, value<0/1(hex), value>0/1(hex)
  condtion/1(cond) -> Relational Operator/1
  signal_conditioning/1(BitLength_BeUsed) -> condtion/1(bitL)
  Constant6/1 -> Add4/2
  Add4/1 -> Out1/1
  Merge/1 -> Product/1
  Product/1 -> Add4/1
  Constant5/1 -> Product/2
  value<0/1(Out1) -> Merge/1
  Constant1/1 -> signal_conditioning/1(In1)

== system UXFD_Lib/Custom/CAN/Get_MsgLength ==
  In1 : Inport
  msg_length : S-Function  FunctionName=msg_length_s  SFunctionDeploymentMode=off  EnableBusSupport=off
  Out1 : Outport
  wires:
  msg_length/1 -> Out1/1
  In1/1 -> msg_length/1

== system UXFD_Lib/Custom/CAN/xbackground1 ==

== system UXFD_Lib/Custom/Diagnose/Dem_SetEventStatus ==
  EveSt : Inport
  bEna : Inport  Port=2
  DEM_EventID : Constant  Value=EventID  SampleTime=-1
  Dem_SetEventStatus_Enable : Subsystem
  wires:
  bEna/1 -> Dem_SetEventStatus_Enable/Enable
  EveSt/1 -> Dem_SetEventStatus_Enable/2(EveSt)
  DEM_EventID/1 -> Dem_SetEventStatus_Enable/1(EventID)

== system UXFD_Lib/Custom/Diagnose/Fim_GetFunctionPermission ==
  FIM_EventID : Constant  Value=FunctionID  SampleTime=-1
  Fim_GetFunctionPermission_Asw : S-Function  FunctionName=Fim_GetFunctionPermission_Asw_SF  SFunctionDeploymentMode=off  EnableBusSupport=off  mask(Legacy Function){SFunctionSpec=void Fim_GetFunctionPermission_Asw(uint16 u1, boolean y1[1]), ShowSpec=on}
      mask prompts: ShowSpec "Display function specification"
      mask help:
      | This block allows you to call the legacy functions specified by the following Legacy Code Tool definition:
      | def.SFunctionName = 'Fim_GetFunctionPermission_Asw_SF';
      | def.OutputFcnSpec = 'void Fim_GetFunctionPermission_Asw(uint16 u1, boolean y1[1])';
      | def.HeaderFiles = {'Fim.h'};
      | def.SourceFiles = {'Fim.c'};
      mask Help: <p>This block was generated automatically by the Legacy Code Tool. For detailed help on this tool, call<a href="matlab:legacy_code('help')"> legacy_code('help')</a>.</p>
      mask Callback ShowSpec:
      | if strcmp(get_param(gcbh, 'ShowSpec'), 'on')
      |   set_param(gcbh, 'MaskDisplay', sprintf('fprintf(''%s'');', get_param(gcbh, 'SFunctionSpec')));
      | else
      |   set_param(gcbh, 'MaskDisplay', sprintf('fprintf(''%s'');', get_param(gcbh, 'FunctionName')));
      | end
      mask Display: fprintf('void Fim_GetFunctionPermission_Asw(uint16 u1, boolean y1[1])');
  bPermission : Outport
  wires:
  Fim_GetFunctionPermission_Asw/1 -> bPermission/1
  FIM_EventID/1 -> Fim_GetFunctionPermission_Asw/1

== system UXFD_Lib/Custom/Diagnose/xbackground1 ==

== system UXFD_Lib/Custom/PIN/PIN ADC ==
  Enable : EnablePort
  S-Function : S-Function  FunctionName=Sws_Io_Adc_Get_xxx_S  SFunctionDeploymentMode=off  EnableBusSupport=off
  Value : Outport
  wires:
  S-Function/1 -> Value/1

== system UXFD_Lib/Custom/PIN/PIN DI ==
  Enable : EnablePort
  S-Function : S-Function  FunctionName=Sws_Io_Dio_Get_xxx_S  SFunctionDeploymentMode=off  EnableBusSupport=off
  Value : Outport
  wires:
  S-Function/1 -> Value/1

== system UXFD_Lib/Custom/PIN/PIN DO ==
  In1 : Inport  OutDataTypeStr=boolean
  Enable : EnablePort
  S-Function : S-Function  FunctionName=Sws_Io_Dio_Set_O_S_xxx_S  SFunctionDeploymentMode=off  EnableBusSupport=off
  wires:
  In1/1 -> S-Function/1

== system UXFD_Lib/Custom/PIN/PIN DO1 ==
  In1 : Inport  OutDataTypeStr=int16
  In2 : Inport  Port=2  OutDataTypeStr=uint32
  Enable : EnablePort
  S-Function : S-Function  FunctionName=Sws_Io_Pwm_SetPeriodAndDuty_xxx_S  SFunctionDeploymentMode=off  EnableBusSupport=off
  wires:
  In1/1 -> S-Function/1
  In2/1 -> S-Function/2

== system UXFD_Lib/Custom/PIN/PIN ICU ==
  Enable : EnablePort
  S-Function : S-Function  FunctionName=Sws_Io_Icu_GetDutyCycle_xxx_S  SFunctionDeploymentMode=off  EnableBusSupport=off
  Value : Outport
  wires:
  S-Function/1 -> Value/1

== system UXFD_Lib/Custom/PIN/xbackground1 ==

== system UXFD_Lib/Standard/Bit Operation/GetBitFnc ==
  BitVal : Inport  OutDataTypeStr=uint32
  Bitwise Operator4 : simulink/Logic and Bit Operations/Bitwise Operator  logicop=AND  UseBitMask=off  NumInputPorts=2  BitMask=bin2dec('1111111111111111')  BitMaskRealWorld=Real World Value
  Data Type Conversion2 : DataTypeConversion
  Fcn : Fcn  Expr=2^u
  Getbit_n : Constant  Value=uint8(2)  OutDataTypeStr=single  SampleTime=-1
  Max : Constant  Value=uint8(31)  OutDataTypeStr=single  SampleTime=-1
  Min : Constant  Value=uint8(0)  OutDataTypeStr=single  SampleTime=-1
  Saturation : UXFD_Lib/Standard/Math/Saturation
  Shift Arithmetic4 : ArithShift  BitShiftNumber=GetBitPar  BitShiftDirection=Right
  Out1 : Outport
  wires:
  Bitwise Operator4/1 -> Shift Arithmetic4/1
  Shift Arithmetic4/1 -> Out1/1
  Saturation/1 -> Fcn/1
  Max/1 -> Saturation/2
  Min/1 -> Saturation/3
  BitVal/1 -> Bitwise Operator4/1
  Fcn/1 -> Data Type Conversion2/1
  Getbit_n/1 -> Saturation/1
  Data Type Conversion2/1 -> Bitwise Operator4/2

== system UXFD_Lib/Standard/Bit Operation/SetBitFnc ==
  BitVal : Inport  OutDataTypeStr=boolean
  BitWise : simulink/Logic and Bit Operations/Bitwise Operator  logicop=AND  UseBitMask=on  BitMask=bin2dec('11111111111111111111111111111111')  BitMaskRealWorld=Stored Integer
  Data Type Conversion : DataTypeConversion
  Data Type Conversion1 : DataTypeConversion  RndMeth=Simplest
  Fcn : Fcn  Expr=2^u
  Max : Constant  Value=uint8(31)  OutDataTypeStr=single  SampleTime=-1
  Min : Constant  Value=uint8(0)  OutDataTypeStr=single  SampleTime=-1
  Product : Product  OutDataTypeStr=uint32
      settings: CopyFcn=set_param(gcbh,'ShowName','off');
  Saturation : UXFD_Lib/Standard/Math/Saturation
  Setbit_n : Constant  Value=uint8(5)  OutDataTypeStr=single  SampleTime=-1
  Out : Outport
  wires:
  BitVal/1 -> Data Type Conversion1/1
  BitWise/1 -> Out/1
  Product/1 -> BitWise/1
  Setbit_n/1 -> Saturation/1
  Fcn/1 -> Data Type Conversion/1
  Data Type Conversion/1 -> Product/2
  Data Type Conversion1/1 -> Product/1
  Saturation/1 -> Fcn/1
  Max/1 -> Saturation/2
  Min/1 -> Saturation/3

== system UXFD_Lib/Standard/Calibration/1-D Lookup Table Without Const_Param ==
  note: Lookup Table 1D ( AVLib™ )
  u : Inport  OutDataTypeStr=double
  Curve : Lookup  InputValues=BreakpointData  Table=Table  LookUpMeth=Interpolation-Use End Values  OutDataTypeStr=double
  y : Outport  OutMin=OutMin  OutMax=OutMax
  wires:
  Curve/1 -> y/1
  u/1 -> Curve/1

== system UXFD_Lib/Standard/Calibration/2-D Lookup Table Without Const_Param ==
  note: Lookup Table 2D ( AVLib™ )
  u1 : Inport  OutDataTypeStr=double
  u2 : Inport  Port=2  OutDataTypeStr=double
  Map : Lookup2D  RowIndex=BreakpointData1  ColumnIndex=BreakpointData2  Table=Table  LookUpMeth=Interpolation-Use End Values  OutDataTypeStr=double
  y : Outport  OutMin=OutMin  OutMax=OutMax
  wires:
  Map/1 -> y/1
  u2/1 -> Map/2
  u1/1 -> Map/1

== system UXFD_Lib/Standard/Calibration/OverRide ==
  override_value : Inport
  switch : Inport  Port=2
  input : Inport  Port=3
  Data Type Conversion2 : DataTypeConversion  OutDataTypeStr=boolean
  Switch1 : Switch  Criteria=u2 ~= 0  Threshold=1  RndMeth=Zero  InputSameDT=on
      settings: AttributesFormatString=%<Criteria>
  Out : Outport
  wires:
  Data Type Conversion2/1 -> Switch1/2
  override_value/1 -> Switch1/1
  switch/1 -> Data Type Conversion2/1
  Switch1/1 -> Out/1
  input/1 -> Switch1/3
